simulink model "practice3"  (Simulink 7.9)
settings: Solver=ode45  StartTime=0.0  StopTime=200  RelTol=1e-3
settings Model: Creator=sony  LastModifiedBy=sony

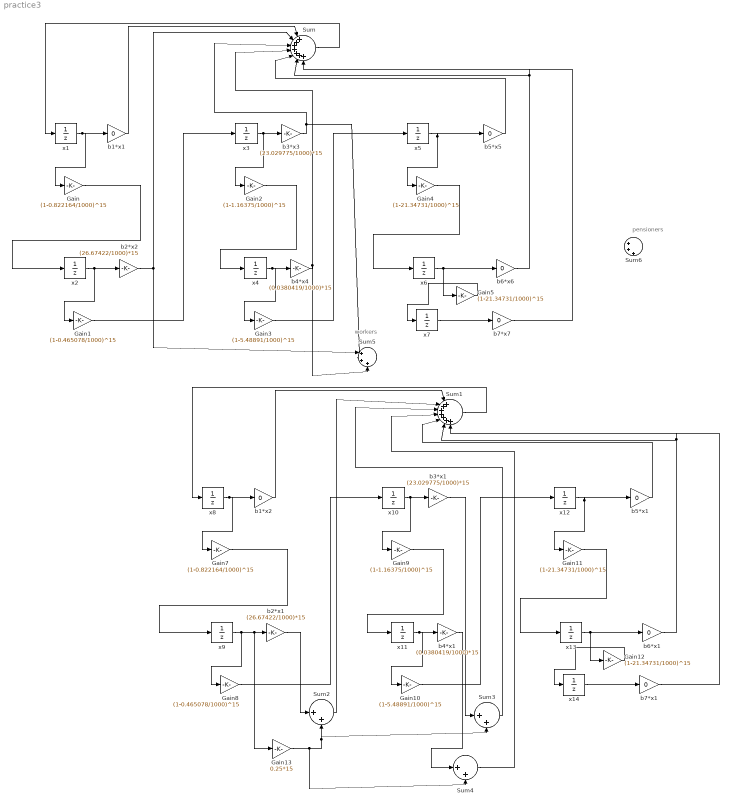
== system practice3 ==
  note: workers
  note: pensioners
  Gain : Gain  Gain=(1-0.822164/1000)^15
  Gain1 : Gain  Gain=(1-0.465078/1000)^15
  Gain10 : Gain  Gain=(1-5.48891/1000)^15
  Gain{4..5,11..12} (4 alike) : Gain  Gain=(1-21.34731/1000)^15
  Gain13 : Gain  Gain=0.25*15
  Gain2 : Gain  Gain=(1-1.16375/1000)^15
  Gain3 : Gain  Gain=(1-5.48891/1000)^15
  Gain7 : Gain  Gain=(1-0.822164/1000)^15
  Gain8 : Gain  Gain=(1-0.465078/1000)^15
  Gain9 : Gain  Gain=(1-1.16375/1000)^15
  Sum : Sum  Inputs=|+++++++
  Sum1 : Sum  Inputs=|+++++++
  Sum2 : Sum  Inputs=|++
  Sum3 : Sum  Inputs=|++
  Sum4 : Sum  Inputs=|++
  Sum5 : Sum  Inputs=|+++
  Sum6 : Sum  Inputs=|+++
  b1*x1 : Gain  Gain=0
  b1*x2 : Gain  Gain=0
  b2*x1 : Gain  Gain=(26.67422/1000)*15
  b2*x2 : Gain  Gain=(26.67422/1000)*15
  b3*x1 : Gain  Gain=(23.029775/1000)*15
  b3*x3 : Gain  Gain=(23.029775/1000)*15
  b4*x1 : Gain  Gain=(0.0380419/1000)*15
  b4*x4 : Gain  Gain=(0.0380419/1000)*15
  b5*x1 : Gain  Gain=0
  b5*x5 : Gain  Gain=0
  b6*x1 : Gain  Gain=0
  b6*x6 : Gain  Gain=0
  b7*x1 : Gain  Gain=0
  b7*x7 : Gain  Gain=0
  x1 : UnitDelay  X0=1494370  SampleTime=15
  x10 : UnitDelay  X0=2474329  SampleTime=15
  x11 : UnitDelay  X0=2142379  SampleTime=15
  x12 : UnitDelay  X0=1626214  SampleTime=15
  x{6..7,13..14} (4 alike) : UnitDelay  X0=665283  SampleTime=15
  x2 : UnitDelay  X0=2075652  SampleTime=15
  x3 : UnitDelay  X0=2474329  SampleTime=15
  x4 : UnitDelay  X0=2142379  SampleTime=15
  x5 : UnitDelay  X0=1626214  SampleTime=15
  x8 : UnitDelay  X0=1494370  SampleTime=15
  x9 : UnitDelay  X0=2075652  SampleTime=15
  wires:
  x1/1 -> Gain/1, b1*x1/1
  Gain/1 -> x2/1
  x2/1 -> b2*x2/1, Gain1/1
  x3/1 -> b3*x3/1, Gain2/1
  x4/1 -> b4*x4/1, Gain3/1
  x5/1 -> b5*x5/1, Gain4/1
  x6/1 -> b6*x6/1, Gain5/1
  Gain1/1 -> x3/1
  Gain2/1 -> x4/1
  Gain3/1 -> x5/1
  Gain4/1 -> x6/1
  b1*x1/1 -> Sum/1
  b2*x2/1 -> Sum/2, Sum5/1
  b3*x3/1 -> Sum/3, Sum5/2
  b4*x4/1 -> Sum/4, Sum5/3
  b5*x5/1 -> Sum/5
  b6*x6/1 -> Sum/6
  x7/1 -> b7*x7/1
  b7*x7/1 -> Sum/7
  Sum/1 -> x1/1
  Gain5/1 -> x7/1
  x8/1 -> Gain7/1, b1*x2/1
  Gain7/1 -> x9/1
  x9/1 -> b2*x1/1, Gain13/1, Gain8/1
  x10/1 -> b3*x1/1, Gain9/1
  x11/1 -> b4*x1/1, Gain10/1
  x12/1 -> b5*x1/1, Gain11/1
  x13/1 -> b6*x1/1, Gain12/1
  Gain8/1 -> x10/1
  Gain9/1 -> x11/1
  Gain10/1 -> x12/1
  Gain11/1 -> x13/1
  b1*x2/1 -> Sum1/1
  b5*x1/1 -> Sum1/5
  b6*x1/1 -> Sum1/6
  x14/1 -> b7*x1/1
  b7*x1/1 -> Sum1/7
  Sum1/1 -> x8/1
  Gain12/1 -> x14/1
  Gain13/1 -> Sum2/2, Sum3/2, Sum4/2
  b2*x1/1 -> Sum2/1
  Sum2/1 -> Sum1/2
  b3*x1/1 -> Sum3/1
  Sum3/1 -> Sum1/3
  b4*x1/1 -> Sum4/1
  Sum4/1 -> Sum1/4
